simulink model "KITTdyn_brake"  (R2018a)
settings: Solver=FixedStepAuto  StartTime=0.0  StopTime=60  FixedStep=0.001  MaxStep=0.01  RelTol=1e-3
undefined symbols (not defined in the file or in its folder): a, b, c, F_ext, m, v0
libraries: simulink x1
settings Model: Creator=Maarteq  LastModifiedBy=Daan
settings CodeAppCC: StateflowObjectComments=on

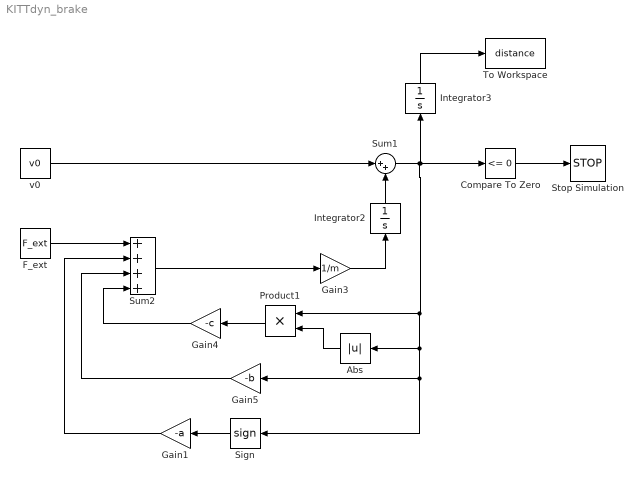
== system KITTdyn_brake ==
  Abs : Abs
  Compare To Zero : simulink/Logic and Bit Operations/Compare To Zero  relop=<=  OutDataTypeStr=boolean
  "F_ext " : Constant  Value=F_ext
  Gain1 : Gain  Gain=-a
  Gain3 : Gain  Gain=1/m
  Gain4 : Gain  Gain=-c
  Gain5 : Gain  Gain=-b
  Integrator2 : Integrator
  Integrator3 : Integrator
  Product1 : Product
  Sign : Signum
  Stop Simulation : Stop
  Sum1 : Sum  Inputs=|++
  Sum2 : Sum  Inputs=++++
  To Workspace : ToWorkspace  VariableName=distance  SaveFormat=Timeseries  SampleTime=-1
  v0 : Constant  Value=v0
  wires:
  v0/1 -> Sum1/1
  Integrator2/1 -> Sum1/2
  Sum1/1 -> Compare To Zero/1, Integrator3/1, Product1/1, Abs/1, Sign/1, Gain5/1
  Product1/1 -> Gain4/1
  Gain4/1 -> Sum2/4
  Gain5/1 -> Sum2/3
  Sum2/1 -> Gain3/1
  "F_ext "/1 -> Sum2/1
  Integrator3/1 -> To Workspace/1
  Abs/1 -> Product1/2
  Gain3/1 -> Integrator2/1
  Sign/1 -> Gain1/1
  Gain1/1 -> Sum2/2
  Compare To Zero/1 -> Stop Simulation/1
